simulink model "p2_1_b_sim"  (R2024b)
settings: Solver=FixedStepAuto  StartTime=0.0  StopTime=150  FixedStep=1e-2  RelTol=1e-3
settings Model: Creator=ruben  LastModifiedBy=ruben

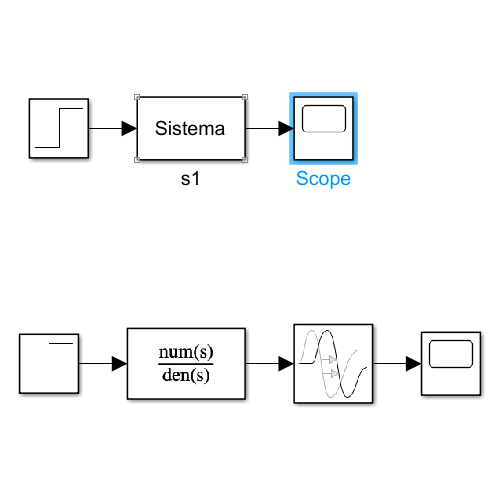
[thumbnail: Simulink's stored preview of the top-level diagram]
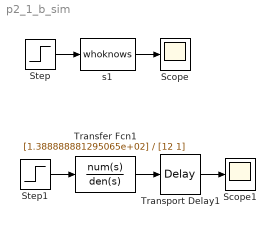
== system p2_1_b_sim ==
  Scope : Scope
  Scope1 : Scope
  Step : Step  SampleTime=0
  Step1 : Step  SampleTime=0
  Transfer Fcn1 : TransferFcn  Numerator=[1.388888881295065e+02]  Denominator=[12 1]
  Transport Delay1 : TransportDelay  DelayTime=6.5
  s1 : M-S-Function  FunctionName=whoknows  Parameters=L, P1, P2, T, R  mask{L=6, P1=2, P2=0, T=1, R=0}
      mask prompts: L "Laboratorio"; P1 "Primer digito del Puesto"; P2 "Segundo digito del Puesto"; T "Tipo de Planta"; R "Ruido"
      mask Display: disp('Sistema')
  wires:
  s1/1 -> Scope/1
  Transport Delay1/1 -> Scope1/1
  Transfer Fcn1/1 -> Transport Delay1/1
  Step/1 -> s1/1
  Step1/1 -> Transfer Fcn1/1
